simulink model "modelirovanieMPY"  (R2020a)
settings: Solver=VariableStepAuto  StartTime=0.0  StopTime=16  RelTol=1e-3
libraries: commseqgen3 x20
settings Model: Creator=Stanislav  LastModifiedBy=Stanislav

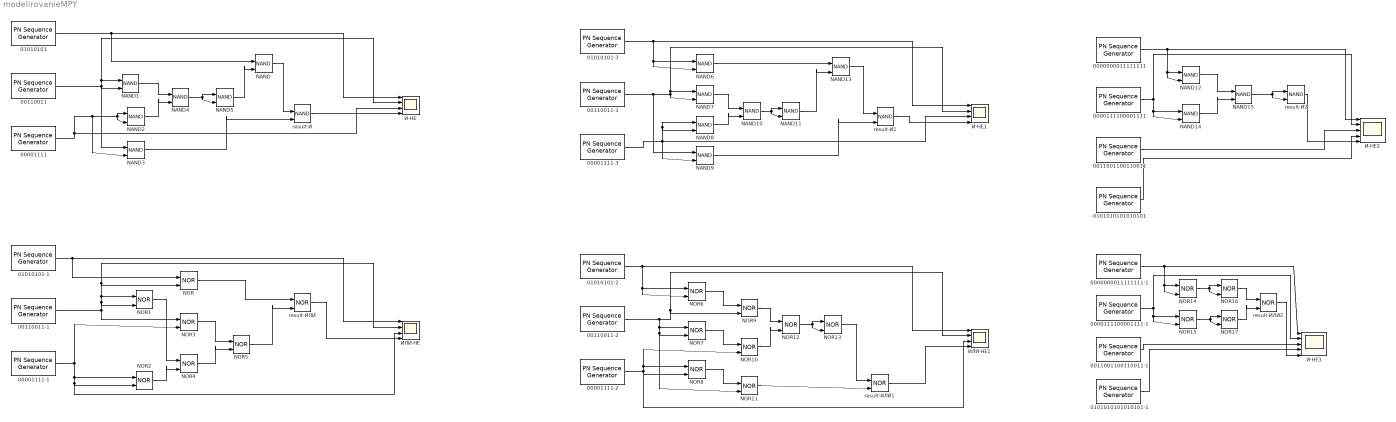
== system modelirovanieMPY ==
  0000000011111111 : commseqgen3/PN Sequence Generator  poly='z^16 + z + 1'  ini_sta=[1 1 1 1 1 1 1 1 0 0 0 0 0 0 0 0]  outBitMaskSource=Dialog parameter  shift=0  outVarSiz=off  maxOutSizeMode=Dialog parameter  maxOutSize=[10 1]  Ts=1  sampPerFrame=1  reset=off  bitPackedOutputs=off  outDataType=double  numPackedBits=8  bitPackDataSigned=off  bitPackedOutDType=double
  0000000011111111-1 : commseqgen3/PN Sequence Generator  poly='z^16 + z + 1'  ini_sta=[1 1 1 1 1 1 1 1 0 0 0 0 0 0 0 0]  outBitMaskSource=Dialog parameter  shift=0  outVarSiz=off  maxOutSizeMode=Dialog parameter  maxOutSize=[10 1]  Ts=1  sampPerFrame=1  reset=off  bitPackedOutputs=off  outDataType=double  numPackedBits=8  bitPackDataSigned=off  bitPackedOutDType=double
  00001111 : commseqgen3/PN Sequence Generator  poly='z^8 + z + 1'  ini_sta=[1 1 1 1 0 0 0 0]  outBitMaskSource=Dialog parameter  shift=0  outVarSiz=off  maxOutSizeMode=Dialog parameter  maxOutSize=[10 1]  Ts=1  sampPerFrame=1  reset=off  bitPackedOutputs=off  outDataType=double  numPackedBits=8  bitPackDataSigned=off  bitPackedOutDType=double
  00001111-1 : commseqgen3/PN Sequence Generator  poly='z^8 + z + 1'  ini_sta=[1 1 1 1 0 0 0 0]  outBitMaskSource=Dialog parameter  shift=0  outVarSiz=off  maxOutSizeMode=Dialog parameter  maxOutSize=[10 1]  Ts=1  sampPerFrame=1  reset=off  bitPackedOutputs=off  outDataType=double  numPackedBits=8  bitPackDataSigned=off  bitPackedOutDType=double
  00001111-2 : commseqgen3/PN Sequence Generator  poly='z^8 + z + 1'  ini_sta=[1 1 1 1 0 0 0 0]  outBitMaskSource=Dialog parameter  shift=0  outVarSiz=off  maxOutSizeMode=Dialog parameter  maxOutSize=[10 1]  Ts=1  sampPerFrame=1  reset=off  bitPackedOutputs=off  outDataType=double  numPackedBits=8  bitPackDataSigned=off  bitPackedOutDType=double
  00001111-3 : commseqgen3/PN Sequence Generator  poly='z^8 + z + 1'  ini_sta=[1 1 1 1 0 0 0 0]  outBitMaskSource=Dialog parameter  shift=0  outVarSiz=off  maxOutSizeMode=Dialog parameter  maxOutSize=[10 1]  Ts=1  sampPerFrame=1  reset=off  bitPackedOutputs=off  outDataType=double  numPackedBits=8  bitPackDataSigned=off  bitPackedOutDType=double
  0000111100001111 : commseqgen3/PN Sequence Generator  poly='z^16 + z + 1'  ini_sta=[1 1 1 1 0 0 0 0 1 1 1 1 0 0 0 0]  outBitMaskSource=Dialog parameter  shift=0  outVarSiz=off  maxOutSizeMode=Dialog parameter  maxOutSize=[10 1]  Ts=1  sampPerFrame=1  reset=off  bitPackedOutputs=off  outDataType=double  numPackedBits=8  bitPackDataSigned=off  bitPackedOutDType=double
  0000111100001111-1 : commseqgen3/PN Sequence Generator  poly='z^16 + z + 1'  ini_sta=[1 1 1 1 0 0 0 0 1 1 1 1 0 0 0 0]  outBitMaskSource=Dialog parameter  shift=0  outVarSiz=off  maxOutSizeMode=Dialog parameter  maxOutSize=[10 1]  Ts=1  sampPerFrame=1  reset=off  bitPackedOutputs=off  outDataType=double  numPackedBits=8  bitPackDataSigned=off  bitPackedOutDType=double
  00110011 : commseqgen3/PN Sequence Generator  poly='z^8 + z + 1'  ini_sta=[1 1 0 0 1 1 0 0]  outBitMaskSource=Dialog parameter  shift=0  outVarSiz=off  maxOutSizeMode=Dialog parameter  maxOutSize=[10 1]  Ts=1  sampPerFrame=1  reset=off  bitPackedOutputs=off  outDataType=double  numPackedBits=8  bitPackDataSigned=off  bitPackedOutDType=double
  00110011-1 : commseqgen3/PN Sequence Generator  poly='z^8 + z + 1'  ini_sta=[1 1 0 0 1 1 0 0]  outBitMaskSource=Dialog parameter  shift=0  outVarSiz=off  maxOutSizeMode=Dialog parameter  maxOutSize=[10 1]  Ts=1  sampPerFrame=1  reset=off  bitPackedOutputs=off  outDataType=double  numPackedBits=8  bitPackDataSigned=off  bitPackedOutDType=double
  00110011-2 : commseqgen3/PN Sequence Generator  poly='z^8 + z + 1'  ini_sta=[1 1 0 0 1 1 0 0]  outBitMaskSource=Dialog parameter  shift=0  outVarSiz=off  maxOutSizeMode=Dialog parameter  maxOutSize=[10 1]  Ts=1  sampPerFrame=1  reset=off  bitPackedOutputs=off  outDataType=double  numPackedBits=8  bitPackDataSigned=off  bitPackedOutDType=double
  00110011-3 : commseqgen3/PN Sequence Generator  poly='z^8 + z + 1'  ini_sta=[1 1 0 0 1 1 0 0]  outBitMaskSource=Dialog parameter  shift=0  outVarSiz=off  maxOutSizeMode=Dialog parameter  maxOutSize=[10 1]  Ts=1  sampPerFrame=1  reset=off  bitPackedOutputs=off  outDataType=double  numPackedBits=8  bitPackDataSigned=off  bitPackedOutDType=double
  0011001100110011 : commseqgen3/PN Sequence Generator  poly='z^16 + z + 1'  ini_sta=[1 1 0 0 1 1 0 0 1 1 0 0 1 1 0 0]  outBitMaskSource=Dialog parameter  shift=0  outVarSiz=off  maxOutSizeMode=Dialog parameter  maxOutSize=[10 1]  Ts=1  sampPerFrame=1  reset=off  bitPackedOutputs=off  outDataType=double  numPackedBits=8  bitPackDataSigned=off  bitPackedOutDType=double
  0011001100110011-1 : commseqgen3/PN Sequence Generator  poly='z^16 + z + 1'  ini_sta=[1 1 0 0 1 1 0 0 1 1 0 0 1 1 0 0]  outBitMaskSource=Dialog parameter  shift=0  outVarSiz=off  maxOutSizeMode=Dialog parameter  maxOutSize=[10 1]  Ts=1  sampPerFrame=1  reset=off  bitPackedOutputs=off  outDataType=double  numPackedBits=8  bitPackDataSigned=off  bitPackedOutDType=double
  01010101 : commseqgen3/PN Sequence Generator  poly='z^8 + z + 1'  ini_sta=[1 0 1 0 1 0 1 0]  outBitMaskSource=Dialog parameter  shift=0  outVarSiz=off  maxOutSizeMode=Dialog parameter  maxOutSize=[10 1]  Ts=1  sampPerFrame=1  reset=off  bitPackedOutputs=off  outDataType=double  numPackedBits=8  bitPackDataSigned=off  bitPackedOutDType=double
  01010101-1 : commseqgen3/PN Sequence Generator  poly='z^8 + z + 1'  ini_sta=[1 0 1 0 1 0 1 0]  outBitMaskSource=Dialog parameter  shift=0  outVarSiz=off  maxOutSizeMode=Dialog parameter  maxOutSize=[10 1]  Ts=1  sampPerFrame=1  reset=off  bitPackedOutputs=off  outDataType=double  numPackedBits=8  bitPackDataSigned=off  bitPackedOutDType=double
  01010101-2 : commseqgen3/PN Sequence Generator  poly='z^8 + z + 1'  ini_sta=[1 0 1 0 1 0 1 0]  outBitMaskSource=Dialog parameter  shift=0  outVarSiz=off  maxOutSizeMode=Dialog parameter  maxOutSize=[10 1]  Ts=1  sampPerFrame=1  reset=off  bitPackedOutputs=off  outDataType=double  numPackedBits=8  bitPackDataSigned=off  bitPackedOutDType=double
  01010101-3 : commseqgen3/PN Sequence Generator  poly='z^8 + z + 1'  ini_sta=[1 0 1 0 1 0 1 0]  outBitMaskSource=Dialog parameter  shift=0  outVarSiz=off  maxOutSizeMode=Dialog parameter  maxOutSize=[10 1]  Ts=1  sampPerFrame=1  reset=off  bitPackedOutputs=off  outDataType=double  numPackedBits=8  bitPackDataSigned=off  bitPackedOutDType=double
  0101010101010101 : commseqgen3/PN Sequence Generator  poly='z^16 + z + 1'  ini_sta=[1 0 1 0 1 0 1 0 1 0 1 0 1 0 1 0]  outBitMaskSource=Dialog parameter  shift=0  outVarSiz=off  maxOutSizeMode=Dialog parameter  maxOutSize=[10 1]  Ts=1  sampPerFrame=1  reset=off  bitPackedOutputs=off  outDataType=double  numPackedBits=8  bitPackDataSigned=off  bitPackedOutDType=double
  0101010101010101-1 : commseqgen3/PN Sequence Generator  poly='z^16 + z + 1'  ini_sta=[1 0 1 0 1 0 1 0 1 0 1 0 1 0 1 0]  outBitMaskSource=Dialog parameter  shift=0  outVarSiz=off  maxOutSizeMode=Dialog parameter  maxOutSize=[10 1]  Ts=1  sampPerFrame=1  reset=off  bitPackedOutputs=off  outDataType=double  numPackedBits=8  bitPackDataSigned=off  bitPackedOutDType=double
  NAND{,1..15} (16 alike) : Logic  Operator=NAND  IconShape=distinctive  AllPortsSameDT=off  OutDataTypeStr=boolean
  NOR{,1..17} (18 alike) : Logic  Operator=NOR  IconShape=distinctive  AllPortsSameDT=off  OutDataTypeStr=boolean
  result-И : Logic  Operator=NAND  IconShape=distinctive  AllPortsSameDT=off  OutDataTypeStr=boolean
  result-И1 : Logic  Operator=NAND  IconShape=distinctive  AllPortsSameDT=off  OutDataTypeStr=boolean
  result-И2 : Logic  Operator=NAND  IconShape=distinctive  AllPortsSameDT=off  OutDataTypeStr=boolean
  result-ИЛИ : Logic  Operator=NOR  IconShape=distinctive  AllPortsSameDT=off  OutDataTypeStr=boolean
  result-ИЛИ1 : Logic  Operator=NOR  IconShape=distinctive  AllPortsSameDT=off  OutDataTypeStr=boolean
  result-ИЛИ2 : Logic  Operator=NOR  IconShape=distinctive  AllPortsSameDT=off  OutDataTypeStr=boolean
  И-НЕ : Scope  NumInputPorts=4
  И-НЕ1 : Scope  NumInputPorts=4
  И-НЕ2 : Scope  NumInputPorts=5
  И-НЕ3 : Scope  NumInputPorts=5
  ИЛИ-НЕ : Scope  NumInputPorts=4
  ИЛИ-НЕ1 : Scope  NumInputPorts=4
  wires:
  01010101/1 -> NAND/1, И-НЕ/1
  00110011/1 -> И-НЕ/2, NAND1/1, NAND3/1, NAND1/2
  00001111/1 -> NAND3/2, NAND2/1, NAND2/2, И-НЕ/3
  NAND1/1 -> NAND4/1
  NAND2/1 -> NAND4/2
  NAND4/1 -> NAND5/2, NAND5/1
  NAND5/1 -> NAND/2
  NAND/1 -> result-И/1
  NAND3/1 -> result-И/2
  result-И/1 -> И-НЕ/4
  01010101-1/1 -> NOR/1, ИЛИ-НЕ/1
  00001111-1/1 -> NOR2/1, NOR2/2, ИЛИ-НЕ/3, NOR3/2
  00110011-1/1 -> NOR3/1, NOR1/2, NOR1/1, NOR/2, ИЛИ-НЕ/2
  result-ИЛИ/1 -> ИЛИ-НЕ/4
  NOR5/1 -> result-ИЛИ/2
  NOR/1 -> result-ИЛИ/1
  NOR2/1 -> NOR4/2
  NOR1/1 -> NOR4/1
  NOR3/1 -> NOR5/1
  NOR4/1 -> NOR5/2
  result-ИЛИ1/1 -> ИЛИ-НЕ1/4
  00110011-2/1 -> NOR7/1, NOR7/2, NOR11/2, NOR9/2, ИЛИ-НЕ1/2
  00001111-2/1 -> NOR8/2, ИЛИ-НЕ1/3, NOR10/2, NOR8/1
  01010101-2/1 -> NOR6/1, NOR6/2, ИЛИ-НЕ1/1
  01010101-3/1 -> NAND6/2, NAND6/1, И-НЕ1/1
  00001111-3/1 -> NAND9/2, NAND8/2, NAND8/1, И-НЕ1/3
  00110011-3/1 -> NAND9/1, NAND7/1, И-НЕ1/2, NAND7/2
  result-И1/1 -> И-НЕ1/4
  NAND9/1 -> result-И1/2
  NAND13/1 -> result-И1/1
  NAND11/1 -> NAND13/2
  NAND6/1 -> NAND13/1
  NAND7/1 -> NAND10/1
  NAND8/1 -> NAND10/2
  NAND10/1 -> NAND11/1, NAND11/2
  NOR12/1 -> NOR13/1, NOR13/2
  NOR13/1 -> result-ИЛИ1/1
  NOR11/1 -> result-ИЛИ1/2
  NOR7/1 -> NOR10/1
  NOR8/1 -> NOR11/1
  NOR6/1 -> NOR9/1
  NOR10/1 -> NOR12/2
  NOR9/1 -> NOR12/1
  0101010101010101/1 -> И-НЕ2/4
  0011001100110011/1 -> И-НЕ2/3
  0000111100001111/1 -> NAND14/2, NAND14/1, И-НЕ2/2
  0000000011111111/1 -> NAND12/2, NAND12/1, И-НЕ2/1
  result-И2/1 -> И-НЕ2/5
  NAND12/1 -> NAND15/1
  NAND14/1 -> NAND15/2
  NAND15/1 -> result-И2/2, result-И2/1
  0011001100110011-1/1 -> И-НЕ3/3
  0000000011111111-1/1 -> NOR14/2, NOR14/1, И-НЕ3/1
  0101010101010101-1/1 -> И-НЕ3/4
  0000111100001111-1/1 -> NOR15/2, NOR15/1, И-НЕ3/2
  result-ИЛИ2/1 -> И-НЕ3/5
  NOR17/1 -> result-ИЛИ2/2
  NOR16/1 -> result-ИЛИ2/1
  NOR14/1 -> NOR16/2, NOR16/1
  NOR15/1 -> NOR17/2, NOR17/1
